simulink subsystem "Channel"  (R2022b)
settings: Solver=VariableStepAuto  StartTime=0.0  StopTime=10.0  RelTol=1e-3
undefined symbols (not defined in the file): channel_cutoff_frequency, time_precision
settings Model: Creator=Ali-Laptop  LastModifiedBy=Ali-Laptop

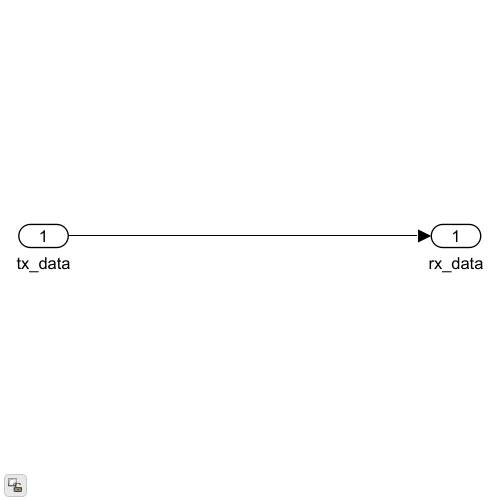
[thumbnail: Simulink's stored preview of the top-level diagram]
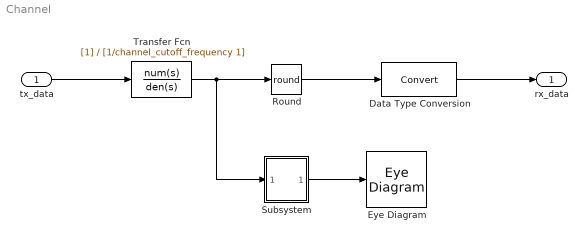
== system Channel ==
  tx_data : Inport
  Data Type Conversion : DataTypeConversion  SaturateOnIntegerOverflow=off  RndMeth=Floor
  Eye Diagram : EyeDiagram
  Round : Rounding  Operator=round
  Subsystem : Subsystem
  Transfer Fcn : TransferFcn  Denominator=[1/channel_cutoff_frequency 1]
  rx_data : Outport
  wires:
  Transfer Fcn/1 -> Round/1, Subsystem/1(In1)
  Data Type Conversion/1 -> rx_data/1
  tx_data/1 -> Transfer Fcn/1
  Round/1 -> Data Type Conversion/1
  Subsystem/1(Out1) -> Eye Diagram/1

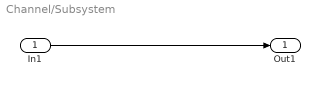
== system Channel/Subsystem ==
  In1 : Inport
  Out1 : Outport  SampleTime=time_precision
  wires:
  In1/1 -> Out1/1
